simulink model "ADCtoDACloopback370"  (R2015b)
settings: Solver=VariableStepAuto  StartTime=0.0  StopTime=10.0  RelTol=1e-3
undefined symbols (not defined in the file): AXI4, fClk, Lite
libraries: xbsIndex_r4 x61
settings Model: Creator=sebek  LastModifiedBy=ulegat

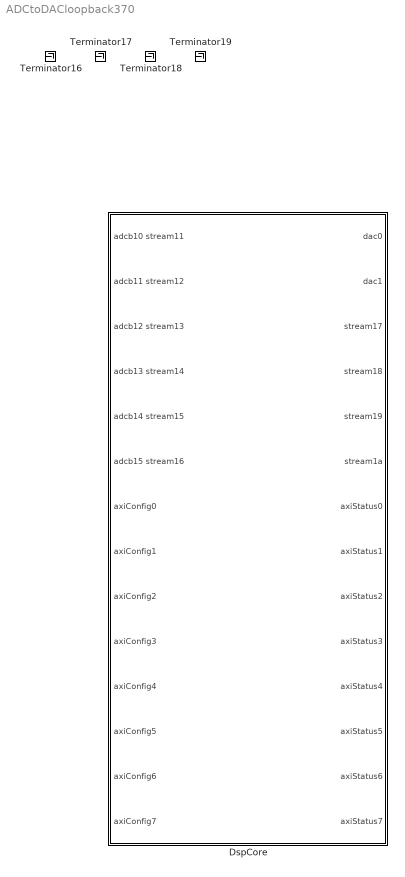
== system ADCtoDACloopback370 ==
  DspCore : Subsystem
  Terminator{16..19} (4 alike) : Terminator

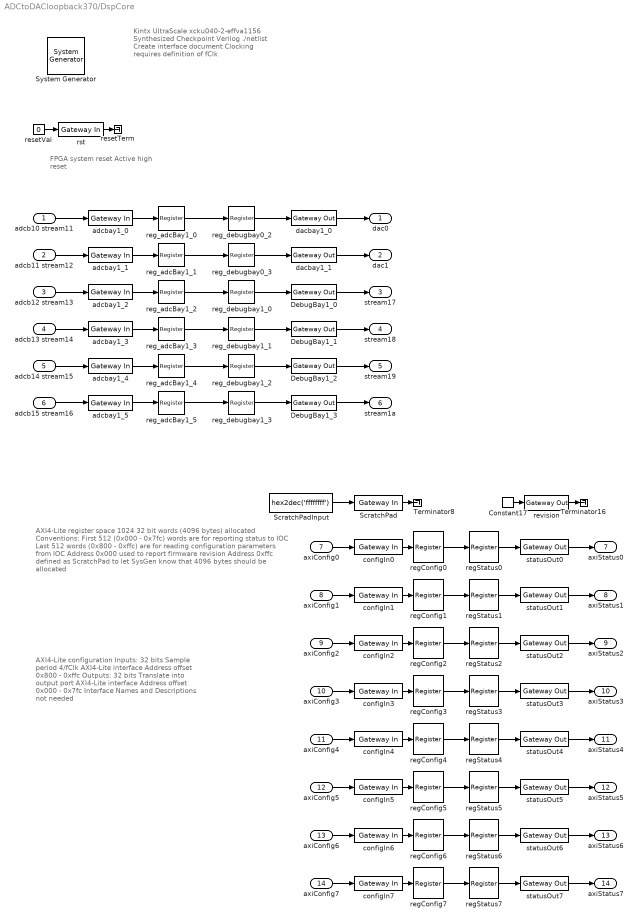
== system ADCtoDACloopback370/DspCore ==
  note: AXI4-Lite configuration
      | Inputs:
      | 32 bits
      | Sample period 4/fClk
      | AXI4-Lite interface
      | Address offset 0x800 - 0xffc
      | Outputs:
      | 32 bits
      | Translate into output port
      | AXI4-Lite interface
      | Address offset 0x000 - 0x7fc
      | Interface Names and Descriptions not needed
  note: AXI4-Lite register space
      | 1024 32 bit words (4096 bytes) allocated
      | Conventions:
      | First 512 (0x000 - 0x7fc) words are for reporting status to IOC
      | Last 512 words (0x800 - 0xffc) are for reading configuration
      | parameters from IOC
      | Address 0x000 used to report firmware revision
      | Address 0xffc defined as ScratchPad to let SysGen know that
      | 4096 bytes should be allocated
  note: Kintx UltraScale xcku040-2-effva1156
      | Synthesized Checkpoint
      | Verilog
      | ./netlist
      | Create interface document
      | Clocking requires definition of fClk
  note: FPGA system reset
      | Active high reset
  adcb10 stream11 : Inport
  adcb11 stream12 : Inport  Port=2
  adcb12 stream13 : Inport  Port=3
  adcb13 stream14 : Inport  Port=4
  adcb14 stream15 : Inport  Port=5
  adcb15 stream16 : Inport  Port=6
  axiConfig0 : Inport  Port=7
  axiConfig1 : Inport  Port=8
  axiConfig2 : Inport  Port=9
  axiConfig3 : Inport  Port=10
  axiConfig4 : Inport  Port=11
  axiConfig5 : Inport  Port=12
  axiConfig6 : Inport  Port=13
  axiConfig7 : Inport  Port=14
  " System Generator" : xbsIndex_r4/ System Generator  Tag=genX  xilinxfamily=kintexu  part=xcku040  speed=-2-e  package=ffva1156  synthesis_tool=Vivado  clock_wrapper=Clock Enables  directory=./netlist  proj_type=Vivado  Synth_file=Vivado Synthesis Defaults  Impl_file=Vivado Implementation Defaults  testbench=off  simulink_period=1/fClk  sysclk_period=1/fClk*1e9  dcm_input_clock_period=10  incr_netlist=off  trim_vbits=Everywhere in SubSystem  dbl_ovrd=According to Block Masks  core_generation=According to Block Masks  run_coregen=off  deprecated_control=off  eval_field=0  block_type=sysgen
  Constant17 : xbsIndex_r4/Constant  const=1  gui_display_data_type=Fixed-point  arith_type=Unsigned  n_bits=32  bin_pt=0  preci_type=Single  exp_width=8  frac_width=24  explicit_period=off  period=1  equ=P=C  opselect=C  inp2=PCIN>>17  opr=+  inp1=P  carry=CIN  dbl_ovrd=off  block_type=constant
  DebugBay1_{0..3} (4 alike) : xbsIndex_r4/Gateway Out  inherit_from_input=on  hdl_port=on  rows=1  columns=1  UseAsDAC=off  DACChannel='1'  interface=None  automatic_assignment=on  address_offset=hex2dec('00')  intf_name=''  intf_description=''  timing_constraint=None  locs_specified=off  LOCs={}  io_standard={}  block_type=gatewayout
  ScratchPad : xbsIndex_r4/Gateway In  gui_display_data_type=Fixed-point  arith_type=Unsigned  n_bits=32  bin_pt=0  preci_type=Single  exp_width=8  frac_width=24  rows=1  columns=1  quantization="Round  (unbiased: +/- Inf)"  overflow=Saturate  period=1  UseAsADC=off  ADCChannel='1'  interface=AXI4-Lite  automatic_assignment=off  address_offset=hex2dec('0ffc')  intf_name=''  intf_description=''  default_value=0  timing_constraint=None  locs_specified=off  LOCs={}  io_standard={}  inherit_from_input=off  hdl_port=on  dbl_ovrd=off  block_type=gatewayin
  ScratchPadInput : Constant  Value=hex2dec('ffffffff')  OutDataTypeStr=uint32
  Terminator16 : Terminator
  Terminator8 : Terminator
  adcbay1_{0..5} (6 alike) : xbsIndex_r4/Gateway In  gui_display_data_type=Fixed-point  arith_type="Signed  (2's comp)"  n_bits=16  bin_pt=0  preci_type=Single  exp_width=8  frac_width=24  rows=1  columns=1  quantization="Round  (unbiased: +/- Inf)"  overflow=Saturate  period=1/fClk  UseAsADC=off  ADCChannel='1'  interface=None  automatic_assignment=on  address_offset=hex2dec('00')  intf_name=''  intf_description=''  default_value=0  timing_constraint=None  locs_specified=off  LOCs={}  io_standard={}  inherit_from_input=off  hdl_port=on  dbl_ovrd=off  block_type=gatewayin
  configIn0 : xbsIndex_r4/Gateway In  gui_display_data_type=Fixed-point  arith_type="Signed  (2's comp)"  n_bits=32  bin_pt=0  preci_type=Single  exp_width=8  frac_width=24  rows=1  columns=1  quantization="Round  (unbiased: +/- Inf)"  overflow=Saturate  period=4/fClk  UseAsADC=off  ADCChannel='1'  interface=AXI4-Lite  automatic_assignment=off  address_offset=hex2dec('800')  intf_name=''  intf_description=''  default_value=0  timing_constraint=None  locs_specified=off  LOCs={}  io_standard={}  inherit_from_input=off  hdl_port=on  dbl_ovrd=off  block_type=gatewayin
  configIn1 : xbsIndex_r4/Gateway In  gui_display_data_type=Fixed-point  arith_type="Signed  (2's comp)"  n_bits=32  bin_pt=0  preci_type=Single  exp_width=8  frac_width=24  rows=1  columns=1  quantization="Round  (unbiased: +/- Inf)"  overflow=Saturate  period=4/fClk  UseAsADC=off  ADCChannel='1'  interface=AXI4-Lite  automatic_assignment=off  address_offset=hex2dec('804')  intf_name=''  intf_description=''  default_value=0  timing_constraint=None  locs_specified=off  LOCs={}  io_standard={}  inherit_from_input=off  hdl_port=on  dbl_ovrd=off  block_type=gatewayin
  configIn2 : xbsIndex_r4/Gateway In  gui_display_data_type=Fixed-point  arith_type="Signed  (2's comp)"  n_bits=32  bin_pt=0  preci_type=Single  exp_width=8  frac_width=24  rows=1  columns=1  quantization="Round  (unbiased: +/- Inf)"  overflow=Saturate  period=4/fClk  UseAsADC=off  ADCChannel='1'  interface=AXI4-Lite  automatic_assignment=off  address_offset=hex2dec('808')  intf_name=''  intf_description=''  default_value=0  timing_constraint=None  locs_specified=off  LOCs={}  io_standard={}  inherit_from_input=off  hdl_port=on  dbl_ovrd=off  block_type=gatewayin
  configIn3 : xbsIndex_r4/Gateway In  gui_display_data_type=Fixed-point  arith_type="Signed  (2's comp)"  n_bits=32  bin_pt=0  preci_type=Single  exp_width=8  frac_width=24  rows=1  columns=1  quantization="Round  (unbiased: +/- Inf)"  overflow=Saturate  period=4/fClk  UseAsADC=off  ADCChannel='1'  interface=AXI4-Lite  automatic_assignment=off  address_offset=hex2dec('80C')  intf_name=''  intf_description=''  default_value=0  timing_constraint=None  locs_specified=off  LOCs={}  io_standard={}  inherit_from_input=off  hdl_port=on  dbl_ovrd=off  block_type=gatewayin
  configIn4 : xbsIndex_r4/Gateway In  gui_display_data_type=Fixed-point  arith_type="Signed  (2's comp)"  n_bits=32  bin_pt=0  preci_type=Single  exp_width=8  frac_width=24  rows=1  columns=1  quantization="Round  (unbiased: +/- Inf)"  overflow=Saturate  period=4/fClk  UseAsADC=off  ADCChannel='1'  interface=AXI4-Lite  automatic_assignment=off  address_offset=hex2dec('810')  intf_name=''  intf_description=''  default_value=0  timing_constraint=None  locs_specified=off  LOCs={}  io_standard={}  inherit_from_input=off  hdl_port=on  dbl_ovrd=off  block_type=gatewayin
  configIn5 : xbsIndex_r4/Gateway In  gui_display_data_type=Fixed-point  arith_type="Signed  (2's comp)"  n_bits=32  bin_pt=0  preci_type=Single  exp_width=8  frac_width=24  rows=1  columns=1  quantization="Round  (unbiased: +/- Inf)"  overflow=Saturate  period=4/fClk  UseAsADC=off  ADCChannel='1'  interface=AXI4-Lite  automatic_assignment=off  address_offset=hex2dec('814')  intf_name=''  intf_description=''  default_value=0  timing_constraint=None  locs_specified=off  LOCs={}  io_standard={}  inherit_from_input=off  hdl_port=on  dbl_ovrd=off  block_type=gatewayin
  configIn6 : xbsIndex_r4/Gateway In  gui_display_data_type=Fixed-point  arith_type="Signed  (2's comp)"  n_bits=32  bin_pt=0  preci_type=Single  exp_width=8  frac_width=24  rows=1  columns=1  quantization="Round  (unbiased: +/- Inf)"  overflow=Saturate  period=4/fClk  UseAsADC=off  ADCChannel='1'  interface=AXI4-Lite  automatic_assignment=off  address_offset=hex2dec('818')  intf_name=''  intf_description=''  default_value=0  timing_constraint=None  locs_specified=off  LOCs={}  io_standard={}  inherit_from_input=off  hdl_port=on  dbl_ovrd=off  block_type=gatewayin
  configIn7 : xbsIndex_r4/Gateway In  gui_display_data_type=Fixed-point  arith_type="Signed  (2's comp)"  n_bits=32  bin_pt=0  preci_type=Single  exp_width=8  frac_width=24  rows=1  columns=1  quantization="Round  (unbiased: +/- Inf)"  overflow=Saturate  period=4/fClk  UseAsADC=off  ADCChannel='1'  interface=AXI4-Lite  automatic_assignment=off  address_offset=hex2dec('81C')  intf_name=''  intf_description=''  default_value=0  timing_constraint=None  locs_specified=off  LOCs={}  io_standard={}  inherit_from_input=off  hdl_port=on  dbl_ovrd=off  block_type=gatewayin
  dacbay1_0 : xbsIndex_r4/Gateway Out  inherit_from_input=off  hdl_port=on  rows=1  columns=1  UseAsDAC=off  DACChannel='1'  interface=None  automatic_assignment=on  address_offset=hex2dec('00')  intf_name=''  intf_description=''  timing_constraint=None  locs_specified=off  LOCs={}  io_standard={}  block_type=gatewayout
  dacbay1_1 : xbsIndex_r4/Gateway Out  inherit_from_input=off  hdl_port=on  rows=1  columns=1  UseAsDAC=off  DACChannel='1'  interface=None  automatic_assignment=on  address_offset=hex2dec('00')  intf_name=''  intf_description=''  timing_constraint=None  locs_specified=off  LOCs={}  io_standard={}  block_type=gatewayout
  regConfig{0..7} (8 alike) : xbsIndex_r4/Register  init=0  rst=off  en=off  dbl_ovrd=off  block_type=register
  regStatus{0..7} (8 alike) : xbsIndex_r4/Register  init=0  rst=off  en=off  dbl_ovrd=off  block_type=register
  reg_adcBay1_{0..5} (6 alike) : xbsIndex_r4/Register  init=0  rst=off  en=off  dbl_ovrd=off  block_type=register
  reg_debugbay0_2 : xbsIndex_r4/Register  init=0  rst=off  en=off  dbl_ovrd=off  block_type=register
  reg_debugbay0_3 : xbsIndex_r4/Register  init=0  rst=off  en=off  dbl_ovrd=off  block_type=register
  reg_debugbay1_{0..3} (4 alike) : xbsIndex_r4/Register  init=0  rst=off  en=off  dbl_ovrd=off  block_type=register
  resetTerm : Terminator
  resetVal : Constant  Value=0
  revision : xbsIndex_r4/Gateway Out  inherit_from_input=off  hdl_port=on  rows=1  columns=1  UseAsDAC=off  DACChannel='1'  interface=AXI4-Lite  automatic_assignment=off  address_offset=hex2dec('000')  intf_name=''  intf_description=''  timing_constraint=None  locs_specified=off  LOCs={}  io_standard={}  block_type=gatewayout
  rst : xbsIndex_r4/Gateway In  gui_display_data_type=Boolean  arith_type=Boolean  n_bits=16  bin_pt=14  preci_type=Single  exp_width=8  frac_width=24  rows=1  columns=1  quantization="Round  (unbiased: +/- Inf)"  overflow=Saturate  period=1/fClk  UseAsADC=off  ADCChannel='1'  interface=None  automatic_assignment=on  address_offset=hex2dec('00')  intf_name=''  intf_description=''  default_value=0  timing_constraint=None  locs_specified=off  LOCs={}  io_standard={}  inherit_from_input=off  hdl_port=on  dbl_ovrd=off  block_type=gatewayin
  statusOut0 : xbsIndex_r4/Gateway Out  inherit_from_input=off  hdl_port=on  rows=1  columns=1  UseAsDAC=off  DACChannel='1'  interface=AXI4-Lite  automatic_assignment=off  address_offset=hex2dec('004')  intf_name=''  intf_description=''  timing_constraint=None  locs_specified=off  LOCs={}  io_standard={}  block_type=gatewayout
  statusOut1 : xbsIndex_r4/Gateway Out  inherit_from_input=off  hdl_port=on  rows=1  columns=1  UseAsDAC=off  DACChannel='1'  interface=AXI4-Lite  automatic_assignment=off  address_offset=hex2dec('008')  intf_name=''  intf_description=''  timing_constraint=None  locs_specified=off  LOCs={}  io_standard={}  block_type=gatewayout
  statusOut2 : xbsIndex_r4/Gateway Out  inherit_from_input=off  hdl_port=on  rows=1  columns=1  UseAsDAC=off  DACChannel='1'  interface=AXI4-Lite  automatic_assignment=off  address_offset=hex2dec('00c')  intf_name=''  intf_description=''  timing_constraint=None  locs_specified=off  LOCs={}  io_standard={}  block_type=gatewayout
  statusOut3 : xbsIndex_r4/Gateway Out  inherit_from_input=off  hdl_port=on  rows=1  columns=1  UseAsDAC=off  DACChannel='1'  interface=AXI4-Lite  automatic_assignment=off  address_offset=hex2dec('010')  intf_name=''  intf_description=''  timing_constraint=None  locs_specified=off  LOCs={}  io_standard={}  block_type=gatewayout
  statusOut4 : xbsIndex_r4/Gateway Out  inherit_from_input=off  hdl_port=on  rows=1  columns=1  UseAsDAC=off  DACChannel='1'  interface=AXI4-Lite  automatic_assignment=off  address_offset=hex2dec('014')  intf_name=''  intf_description=''  timing_constraint=None  locs_specified=off  LOCs={}  io_standard={}  block_type=gatewayout
  statusOut5 : xbsIndex_r4/Gateway Out  inherit_from_input=off  hdl_port=on  rows=1  columns=1  UseAsDAC=off  DACChannel='1'  interface=AXI4-Lite  automatic_assignment=off  address_offset=hex2dec('018')  intf_name=''  intf_description=''  timing_constraint=None  locs_specified=off  LOCs={}  io_standard={}  block_type=gatewayout
  statusOut6 : xbsIndex_r4/Gateway Out  inherit_from_input=off  hdl_port=on  rows=1  columns=1  UseAsDAC=off  DACChannel='1'  interface=AXI4-Lite  automatic_assignment=off  address_offset=hex2dec('01c')  intf_name=''  intf_description=''  timing_constraint=None  locs_specified=off  LOCs={}  io_standard={}  block_type=gatewayout
  statusOut7 : xbsIndex_r4/Gateway Out  inherit_from_input=off  hdl_port=on  rows=1  columns=1  UseAsDAC=off  DACChannel='1'  interface=AXI4-Lite  automatic_assignment=off  address_offset=hex2dec('020')  intf_name=''  intf_description=''  timing_constraint=None  locs_specified=off  LOCs={}  io_standard={}  block_type=gatewayout
  dac0 : Outport
  dac1 : Outport  Port=2
  stream17 : Outport  Port=3
  stream18 : Outport  Port=4
  stream19 : Outport  Port=5
  stream1a : Outport  Port=6
  axiStatus0 : Outport  Port=7
  axiStatus1 : Outport  Port=8
  axiStatus2 : Outport  Port=9
  axiStatus3 : Outport  Port=10
  axiStatus4 : Outport  Port=11
  axiStatus5 : Outport  Port=12
  axiStatus6 : Outport  Port=13
  axiStatus7 : Outport  Port=14
  wires:
  reg_adcBay1_0/1 -> reg_debugbay0_2/1
  adcbay1_0/1 -> reg_adcBay1_0/1
  reg_adcBay1_1/1 -> reg_debugbay0_3/1
  adcbay1_1/1 -> reg_adcBay1_1/1
  reg_adcBay1_2/1 -> reg_debugbay1_0/1
  adcbay1_2/1 -> reg_adcBay1_2/1
  reg_adcBay1_3/1 -> reg_debugbay1_1/1
  adcbay1_3/1 -> reg_adcBay1_3/1
  reg_adcBay1_4/1 -> reg_debugbay1_2/1
  adcbay1_4/1 -> reg_adcBay1_4/1
  reg_adcBay1_5/1 -> reg_debugbay1_3/1
  adcbay1_5/1 -> reg_adcBay1_5/1
  ScratchPad/1 -> Terminator8/1
  dacbay1_1/1 -> dac1/1
  dacbay1_0/1 -> dac0/1
  adcb15 stream16/1 -> adcbay1_5/1
  adcb12 stream13/1 -> adcbay1_2/1
  adcb10 stream11/1 -> adcbay1_0/1
  adcb11 stream12/1 -> adcbay1_1/1
  DebugBay1_0/1 -> stream17/1
  DebugBay1_1/1 -> stream18/1
  DebugBay1_2/1 -> stream19/1
  DebugBay1_3/1 -> stream1a/1
  axiConfig0/1 -> configIn0/1
  configIn0/1 -> regConfig0/1
  statusOut0/1 -> axiStatus0/1
  axiConfig1/1 -> configIn1/1
  configIn1/1 -> regConfig1/1
  statusOut1/1 -> axiStatus1/1
  axiConfig2/1 -> configIn2/1
  configIn2/1 -> regConfig2/1
  statusOut2/1 -> axiStatus2/1
  axiConfig3/1 -> configIn3/1
  configIn3/1 -> regConfig3/1
  statusOut3/1 -> axiStatus3/1
  revision/1 -> Terminator16/1
  Constant17/1 -> revision/1
  resetVal/1 -> rst/1
  rst/1 -> resetTerm/1
  adcb14 stream15/1 -> adcbay1_4/1
  adcb13 stream14/1 -> adcbay1_3/1
  reg_debugbay1_3/1 -> DebugBay1_3/1
  reg_debugbay1_0/1 -> DebugBay1_0/1
  reg_debugbay1_1/1 -> DebugBay1_1/1
  reg_debugbay1_2/1 -> DebugBay1_2/1
  regStatus0/1 -> statusOut0/1
  regConfig0/1 -> regStatus0/1
  regConfig1/1 -> regStatus1/1
  regConfig2/1 -> regStatus2/1
  regConfig3/1 -> regStatus3/1
  regStatus3/1 -> statusOut3/1
  regStatus2/1 -> statusOut2/1
  regStatus1/1 -> statusOut1/1
  axiConfig4/1 -> configIn4/1
  configIn4/1 -> regConfig4/1
  statusOut4/1 -> axiStatus4/1
  axiConfig5/1 -> configIn5/1
  configIn5/1 -> regConfig5/1
  statusOut5/1 -> axiStatus5/1
  axiConfig6/1 -> configIn6/1
  configIn6/1 -> regConfig6/1
  statusOut6/1 -> axiStatus6/1
  axiConfig7/1 -> configIn7/1
  configIn7/1 -> regConfig7/1
  statusOut7/1 -> axiStatus7/1
  regStatus4/1 -> statusOut4/1
  regConfig4/1 -> regStatus4/1
  regConfig5/1 -> regStatus5/1
  regConfig6/1 -> regStatus6/1
  regConfig7/1 -> regStatus7/1
  regStatus7/1 -> statusOut7/1
  regStatus6/1 -> statusOut6/1
  regStatus5/1 -> statusOut5/1
  ScratchPadInput/1 -> ScratchPad/1
  reg_debugbay0_2/1 -> dacbay1_0/1
  reg_debugbay0_3/1 -> dacbay1_1/1
